simulink model "parameter_State_estimation_sim_model"  (R2018b)
settings: Solver=VariableStepAuto  StartTime=0.0  StopTime=10.0  RelTol=1e-3
libraries: simulink x2, sharedTrackingLibrary x1
settings Model: Creator=chpark  LastModifiedBy=chpark

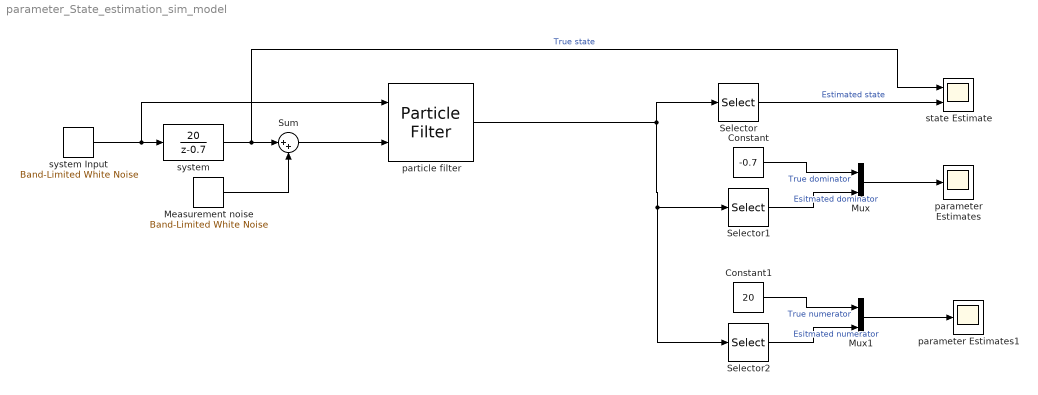
== system parameter_State_estimation_sim_model ==
  Constant : Constant  Value=-0.7
  Constant1 : Constant  Value=20
  Measurement noise : simulink/Sources/Band-Limited White Noise  Cov=1  Ts=1  seed=[23342]
  Mux : Mux  Inputs=2
  Mux1 : Mux  Inputs=2
  Selector : Selector  InputPortWidth=3  IndexOptions=Index vector (dialog)  Indices=[1]  OutputSizes=1
  Selector1 : Selector  InputPortWidth=3  IndexOptions=Index vector (dialog)  Indices=[2]  OutputSizes=1
  Selector2 : Selector  InputPortWidth=3  IndexOptions=Index vector (dialog)  Indices=[3]  OutputSizes=1
  Sum : Sum  Inputs=|++
  parameter Estimates : Scope
  parameter Estimates1 : Scope
  particle filter : sharedTrackingLibrary/Particle Filter  StateTransitionFcn=PF_StateTransitionFcn  HasStateTransitionFcnExtraArgument=1  NumberOfParticles=10000  InitialDistribution=Gaussian  InitialMean=[0;0;0]  InitialCovariance=diag([1e1 5 1e3])  InitialStateBounds=[-3 3; -3 3]  InitialParticles=[]  InitialWeights=[]  CircularVariables=0  StateOrientation=Column  MeasurementLikelihoodFcn1=PF_MeasurementFcn  HasMeasurementEnablePort1=off  HasMeasurementFcnExtraArgument1=0  HasMeasurementEnablePort2=off  HasMeasurementFcnExtraArgument2=0  HasMeasurementEnablePort3=off  HasMeasurementFcnExtraArgument3=0  HasMeasurementEnablePort4=off  HasMeasurementFcnExtraArgument4=0  HasMeasurementEnablePort5=off  HasMeasurementFcnExtraArgument5=0  ResamplingMethod=Multinomial  TriggerMethod=Ratio  MinEffectiveParticleRatio=0.5  SamplingInterval=1  Randomness=Repeatable  Seed=0  StateEstimationMethod=Mean  OutputParticles=off  OutputWeights=off  OutputStateCovariance=off  UseCurrentEstimator=on  EnableMultirate=off  StateTransitionFcnSampleTime=1  MeasurementLikelihoodFcn1SampleTime=1  MeasurementLikelihoodFcn2SampleTime=1  MeasurementLikelihoodFcn3SampleTime=1  MeasurementLikelihoodFcn4SampleTime=1  MeasurementLikelihoodFcn5SampleTime=1  DataType=double  SampleTime=1  NumberOfMeasurements=1
      settings: SourceProductName=Control System Toolbox  SourceProductBaseCode=CT
  state Estimate : Scope  NumInputPorts=2
  system : DiscreteTransferFcn  Numerator=[0 20]  Denominator=[1 -0.7]
  system Input : simulink/Sources/Band-Limited White Noise  Cov=10  Ts=1  seed=[23340]
  wires:
  system Input/1 -> particle filter/1, system/1
  system/1 -> state Estimate/1, Sum/1  "True state"
  Measurement noise/1 -> Sum/2
  Selector/1 -> state Estimate/2  "Estimated state"
  particle filter/1 -> Selector/1, Selector2/1, Selector1/1
  Constant/1 -> Mux/1  "True dominator"
  Selector1/1 -> Mux/2  "Esitmated dominator"
  Mux/1 -> parameter Estimates/1
  Constant1/1 -> Mux1/1  "True numerator"
  Selector2/1 -> Mux1/2  "Esitmated numerator"
  Sum/1 -> particle filter/2
  Mux1/1 -> parameter Estimates1/1
